simulink model "h2omnix"  (R2022b)
settings: Solver=VariableStepAuto  StartTime=0.0  StopTime=inf  RelTol=1e-3
libraries: MarineRoboticsLib x2
settings Model: Creator=dnad  LastModifiedBy=dnad

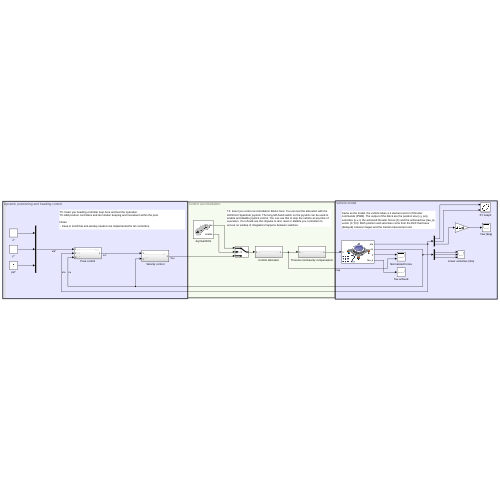
[thumbnail: Simulink's stored preview of the top-level diagram]
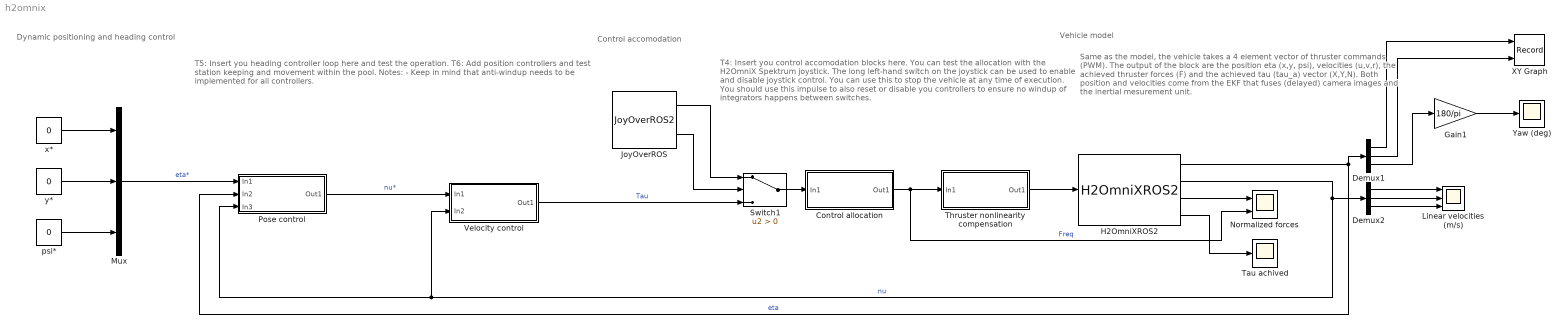
== system h2omnix ==
  note: Control accomodation
  note: T4: Insert you control accomodation blocks here. You can test the allocation with the
      | H2OmniX Spektrum joystick. The long left-hand switch on the joystick can be used to enable and disable joystick control. You can use this to stop the vehicle at any time of execution. You should use this impulse to also reset or disable you controllers to ensure no windup of integrators happens between switches.
  note: Dynamic positioning and heading control
  note: Vehicle model
  note: T5: Insert you heading controller loop here and test the operation.
      | T6: Add position controllers and test station keeping and movement within the pool.
      |
      | Notes:
      |  - Keep in mind that anti-windup needs to be implemented for all controllers.
  note: Same as the model, the vehicle takes a 4 element vector of thruster
      | commands (PWM). The output of the block are the position eta (x,y, psi),
      | velocities (u,v,r), the achieved thruster forces (F) and the achieved tau (tau_a)
      | vector (X,Y,N). Both position and velocities come from the EKF that fuses
      | (delayed) camera images and the inertial mesurement unit.
  Control allocation : Subsystem
  Demux1 : Demux  Outputs=3
  Demux2 : Demux  Outputs=3
  Gain1 : Gain  Gain=180/pi
  H2OmniXROS2 : MarineRoboticsLib/H2OmniXROS2  SystemSampleTime=-1  VariantActivationTime=update diagram  Latency=0  AutoFrameSizeCalculation=off
  JoyOverROS : MarineRoboticsLib/JoyOverROS2  SystemSampleTime=-1  VariantActivationTime=update diagram  Latency=0  AutoFrameSizeCalculation=off
  Linear velocities (m/s) : Scope  NumInputPorts=3
  Mux : Mux  Inputs=3
  Normalized forces : Scope  NumInputPorts=2
  Pose control : Subsystem
  Switch1 : Switch  Criteria=u2 > Threshold  SaturateOnIntegerOverflow=off  InputSameDT=off
  Tau achived : Scope
  Thruster nonlinearity compensation : Subsystem
  Velocity control : Subsystem
  XY Graph : Record  FileSettingsInternal="{\"entries\":[{\"content\":{\"excelSettings\":{\"content\":{},\"type\":\"Streamout.ExcelSettings\"}},\"type\":\"Streamout.FileSettingStorage\",\"uuid\":\"c2ccf2ae-488c-4bcf-8440-ec82bd5a1921\"}],\"packageUris\":[\"http://schema.mathworks.com/mf0/streamout_blocks/R2020a\"],\"version\":\"1.0\"}"  Layout=[1 1]  SignalsInternal="{\"entries\":[{\"content\":{\"signals\":[{\"content\":{\"blockPath\":[\"h2omnix/XY Graph\"],\"channel\":[],\"dimensions\":[1],\"domain\":\"h2omnix/XY Graph\",\"lineColor\":\"#a2142f\",\"plots\":[1],\"port\":1,\"sid\":[],\"signalID\":33,\"signalName\":\"XY Graph:1\"},\"type\":\"RecordBlkView.Signal\",\"uuid\":\"988fb235-ad8a-4eba-9e77-4438b6786f59\"},{\"content\":{\"blockPath\":[\"h2omnix/XY Graph\"],\"channel\":[],\"dimensions\":[1],\"domain\":\"h2omnix/XY Graph\",\"lineColor\":\"#139fff\",\"plots\":[1],\"port\":2,\"sid\":[],\"signalID\":36,\"signalName\":\"XY Graph:2\"},\"type\":\"RecordBlkView.Signal\",\"uuid\":\"17a51127-2417-451c-a370-92b9da37ddba\"}]},\"type\":\"RecordBlkView.InputSignals\",\"uuid\":\"5cbcfa84-bccf-45f4-bb03-fc42fd5fc121\"}],\"packageUris\":[\"http://schema.mathworks.com/mf0/streamout_blocks/R2020a\"],\"version\":\"1.0\"}"  VisualizationBindings="{\"xyplotplugin\":{\"info\":[{\"series\":[{\"bindingParametersList\":[{\"parameter\":\"X-Axis\",\"signalID\":33,\"signalName\":\"XY Graph:1\"},{\"parameter\":\"Y-Axis\",\"signalID\":36,\"signalName\":\"XY Graph:2\"}],\"seriesID\":53718}],\"subplotID\":1}]}}"  CompatibilityTag=XY
  Yaw (deg) : Scope
  psi* : Constant  Value=0
  x* : Constant  Value=0
  y* : Constant  Value=0
  wires:
  Demux2/1 -> Linear velocities (m/s)/1
  H2OmniXROS2/4 -> Tau achived/1
  y*/1 -> Mux/2
  Thruster nonlinearity compensation/1(Out1) -> H2OmniXROS2/1
  H2OmniXROS2/1 -> Demux1/1, Pose control/2(In2)  "eta"
  Control allocation/1(Out1) -> Thruster nonlinearity compensation/1(In1), Normalized forces/2  "Freq"
  psi*/1 -> Mux/3
  H2OmniXROS2/3 -> Normalized forces/1
  Demux1/2 -> XY Graph/2
  H2OmniXROS2/2 -> Pose control/3(In3), Velocity control/2(In2), Demux2/1  "nu"
  Demux1/1 -> XY Graph/1
  Gain1/1 -> Yaw (deg)/1
  Demux1/3 -> Gain1/1
  Pose control/1(Out1) -> Velocity control/1(In1)  "nu*"
  Mux/1 -> Pose control/1(In1)  "eta*"
  Demux2/2 -> Linear velocities (m/s)/2
  x*/1 -> Mux/1
  Demux2/3 -> Linear velocities (m/s)/3
  Switch1/1 -> Control allocation/1(In1)
  JoyOverROS/1 -> Switch1/1
  JoyOverROS/2 -> Switch1/2
  Velocity control/1(Out1) -> Switch1/3  "Tau"

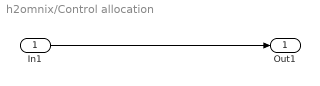
== system h2omnix/Control allocation ==
  In1 : Inport
  Out1 : Outport
  wires:
  In1/1 -> Out1/1

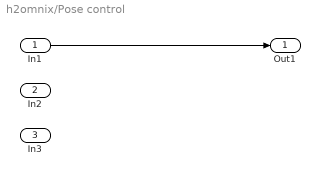
== system h2omnix/Pose control ==
  In1 : Inport
  In2 : Inport  Port=2
  In3 : Inport  Port=3
  Out1 : Outport
  wires:
  In1/1 -> Out1/1

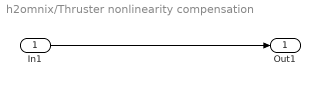
== system h2omnix/Thruster nonlinearity compensation ==
  In1 : Inport
  Out1 : Outport
  wires:
  In1/1 -> Out1/1

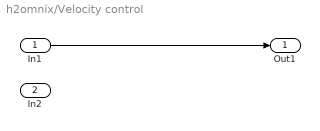
== system h2omnix/Velocity control ==
  In1 : Inport
  In2 : Inport  Port=2
  Out1 : Outport
  wires:
  In1/1 -> Out1/1
